simulink model "VB_RIFKF_GNSS_INS25"  (R2023a)
settings: Solver=FixedStepAuto  StartTime=0  StopTime=500  FixedStep=0.01  RelTol=1e-3
InitFcn:
  | resilient_initNavigation1216;
  | init_param;
undefined symbols (not defined in the file or in its folder): dt, g0, gam0_rad, ISUS_flag, magnitude, p, P0, P0_RIEKF, param, pd0, pe0, phi0_rad, pn0, psi, psi0_rad, state_dim, vd0, ve0, vn0
libraries: simulink_extras x68, dspstat3 x54, sharedtransform x47, simulink x43, matrix_library x9, sharedTrackingLibrary x5, dspfactors x4, aerolibconvert2 x3, aerolibtransform2 x3
(part 12 of 22)

== system VB_RIFKF_GNSS_INS25/No.1_Sensor_Data_Process1/GPS_Data_Process/LLA2NED ==
  note: Vecef2ned
  gps_LLA_rad : Inport
  GPSfixtype : Inport  Port=2
  GPS_Vecef_m/s : Inport  Port=3
  QGC_sensor_reinit : Inport  Port=4
  GPS0 : Inport  Port=5
  Angle Conversion1 : aerolibconvert2/Angle Conversion  IU=deg  OU=rad
  Bus Creator : BusCreator  Inputs=3
  Bus Creator1 : BusCreator  Inputs=3
  Bus Selector : BusSelector  OutputSignals=lon_gps,lat_gps
  Bus Selector1 : BusSelector  OutputSignals=lat_gps,lon_gps,H_gps
  Constant1 : Constant  Value=-90
  Constant4 : Constant  Value=0
  Data Type Conversion{,1..3} (4 alike) : DataTypeConversion  OutDataTypeStr=single  SaturateOnIntegerOverflow=off  RndMeth=Floor
  Demux : Demux  Outputs=3
  Demux1 : Demux  Outputs=3
  Demux3 : Demux  Outputs=3
  Detect Increase : simulink/Logic and Bit Operations/Detect Increase  vinit=0.0  OutDataTypeStr=boolean
  Digital Clock : DigitalClock  SampleTime=0.01
  Direction Cosine Matrix ECEF to NED : aerolibtransform2/Direction Cosine Matrix ECEF to NED  Commented=on
  Divide1 : Product  Inputs=**  Multiplication=Matrix(*)
  Gain : Gain  Gain=-1
  LLA to ECEF Position : LLA2ECEF  R=6378137
  LLA to ECEF Position1 : LLA2ECEF  R=6378137
  MATLAB Function2 : MATLAB Function  TreatAsAtomicUnit=on
  Mux2 : Mux  Inputs=3
  Mux5 : Mux  Inputs=2
  Mux6 : Mux  Inputs=2
  Product : Product  Commented=on  Multiplication=Matrix(*)
  Radians to Degrees{,1..3} (4 alike) : simulink_extras/Transformations/Radians to Degrees
  Radians to Degrees4 : simulink_extras/Transformations/Radians to Degrees  Commented=on
  Rotation Angles to Direction Cosine Matrix : sharedtransform/Rotation Angles to Direction Cosine Matrix  rotationOrder=ZYX  aMode=aMode
  Scope1 : Scope
  Selector2 : Selector  Commented=on  InputPortWidth=3  IndexOptions=Index vector (dialog)  Indices=[1 2]  OutputSizes=1
  Sum : Sum  Inputs=|++
  Sum1 : Sum  Inputs=|+-
  initGPSLLA : MATLAB Function  TreatAsAtomicUnit=on
  "gpsposNEDout " : Outport
  gpsvNEDout : Outport  Port=2
  wires:
  GPSfixtype/1 -> initGPSLLA/2(GPSfixtype)
  Bus Creator1/1 -> "gpsposNEDout "/1, Scope1/1
  Demux3/3 -> Data Type Conversion2/1  "gpspos_D"
  Demux3/2 -> Data Type Conversion1/1  "gpspos_E"
  Demux3/1 -> Data Type Conversion/1  "gpspos_N"
  Bus Creator/1 -> Bus Selector/1, Bus Selector1/1
  Demux/3 -> Bus Creator/3  "H_gps"
  Demux/2 -> Bus Creator/2  "lon_gps"
  Demux/1 -> Bus Creator/1  "lat_gps"
  Demux1/3 -> LLA to ECEF Position1/2
  Mux6/1 -> LLA to ECEF Position1/1
  Mux5/1 -> LLA to ECEF Position/1
  Gain/1 -> Sum/1
  LLA to ECEF Position1/1 -> Sum1/1
  Constant4/1 -> Mux2/3
  Sum1/1 -> Divide1/2
  Demux1/1 -> Radians to Degrees/1
  Mux2/1 -> Rotation Angles to Direction Cosine Matrix/1
  Rotation Angles to Direction Cosine Matrix/1 -> Divide1/1
  Constant1/1 -> Angle Conversion1/1
  LLA to ECEF Position/1 -> Sum1/2
  Demux1/2 -> Radians to Degrees1/1
  Sum/1 -> Mux2/2
  Bus Selector/2 -> Gain/1  "<lat_gps>"
  Bus Selector/1 -> Mux2/1  "<lon_gps>"
  Bus Selector1/1 -> Radians to Degrees2/1  "<lat_gps>"
  Bus Selector1/2 -> Radians to Degrees3/1  "<lon_gps>"
  Bus Selector1/3 -> LLA to ECEF Position/2  "<H_gps>"
  gps_LLA_rad/1 -> initGPSLLA/3(gps_LLA_rad), Selector2/1, Demux1/1
  Radians to Degrees/1 -> Mux6/1
  Radians to Degrees1/1 -> Mux6/2
  QGC_sensor_reinit/1 -> Detect Increase/1
  Data Type Conversion/1 -> Bus Creator1/1  "gpspos_N"
  Data Type Conversion1/1 -> Bus Creator1/2  "gpspos_E"
  Data Type Conversion2/1 -> Bus Creator1/3  "gpspos_D"
  Angle Conversion1/1 -> Sum/2
  Radians to Degrees2/1 -> Mux5/1
  Radians to Degrees3/1 -> Mux5/2
  GPS_Vecef_m/s/1 -> Data Type Conversion3/1, Product/2
  Direction Cosine Matrix ECEF to NED/1 -> Product/1
  Selector2/1 -> Radians to Degrees4/1
  Radians to Degrees4/1 -> Direction Cosine Matrix ECEF to NED/1
  Data Type Conversion3/1 -> gpsvNEDout/1  "gpspos_N"
  Detect Increase/1 -> initGPSLLA/1(QGCinitflag)
  initGPSLLA/1(gpsLLA0_rad) -> Demux/1
  Divide1/1 -> Demux3/1, MATLAB Function2/2(u)
  Digital Clock/1 -> MATLAB Function2/1(t)

== system VB_RIFKF_GNSS_INS25/No.1_Sensor_Data_Process1/GPS_Data_Process/heading_GPS ==
  Vned : Inport
  Atan2 : Trigonometry  Operator=atan2
  Compare To Constant : simulink/Logic and Bit Operations/Compare To Constant  relop=>=  const=0.8  OutDataTypeStr=boolean
  Math Function : Math  Operator=magnitude^2  SignedPower=on
  Moving Average1 : dspstat3/Moving Average  Commented=on  Method=Sliding window  ForgettingFactorPort=off  SpecifyWindowLength=on  WindowLength=10  OverlapLength=9  AllowArbitraryInputLength=off  ForgettingFactor=0.9  SimulateUsing=Code generation
  Scope : Scope  NumInputPorts=2
  Scope1 : Scope
  Selector2 : Selector  InputPortWidth=3  IndexOptions=Index vector (dialog)  Indices=[2]  OutputSizes=1
  Selector3 : Selector  InputPortWidth=3  IndexOptions=Index vector (dialog)  Indices=[1]  OutputSizes=1
  Selector4 : Selector  InputPortWidth=3  IndexOptions=Index vector (dialog)  Indices=[1 2]  OutputSizes=1
  Sqrt : Sqrt
  Sum of Elements : Sum  Inputs=+
  heading_GPS_rad : Outport
  heading_GPS_valid : Outport  Port=2
  wires:
  Selector2/1 -> Atan2/1
  Math Function/1 -> Sum of Elements/1
  Vned/1 -> Selector2/1, Selector4/1, Selector3/1
  Selector3/1 -> Atan2/2
  Sum of Elements/1 -> Sqrt/1
  Selector4/1 -> Math Function/1
  Sqrt/1 -> Compare To Constant/1
  Compare To Constant/1 -> Scope1/1, heading_GPS_valid/1
  Atan2/1 -> Scope/1, Scope/2, heading_GPS_rad/1

== system VB_RIFKF_GNSS_INS25/No.1_Sensor_Data_Process1/IMU_Data_Process/Bias Eliminate ==
  gyro_B_rad/s_ori : Inport
  Data Type Conversion : DataTypeConversion  OutDataTypeStr=single  SaturateOnIntegerOverflow=off  RndMeth=Floor
  Digital Clock : DigitalClock
  Memory : Memory
  Scope : Scope
  Subsystem : Subsystem
  Sum : Sum  Inputs=|+-
  Switch : Switch  Criteria=u2 > Threshold  Threshold=5  SaturateOnIntegerOverflow=off  InputSameDT=off
  Out1 : Outport
  wires:
  Data Type Conversion/1 -> Out1/1
  gyro_B_rad/s_ori/1 -> Subsystem/1(data), Sum/1
  Sum/1 -> Data Type Conversion/1
  Digital Clock/1 -> Switch/2
  Subsystem/1(mean_data) -> Switch/3
  Switch/1 -> Scope/1, Memory/1
  Memory/1 -> Switch/1

== system VB_RIFKF_GNSS_INS25/No.1_Sensor_Data_Process1/IMU_Data_Process/accl_preprocessing2 ==
  note: front-right-dowm
  accl_B_m/s_ori : Inport
  Constant2 : Constant  Value=1/dt  OutDataTypeStr=single
  Constant4 : Constant  Value=1/dt  OutDataTypeStr=single
  Constant6 : Constant  Value=1/dt  OutDataTypeStr=single
  Constant7 : Constant  Value=param.proces.imu_gyro_cutoff_freq  OutDataTypeStr=single
  Demux : Demux  Outputs=3
  MATLAB Function1 : MATLAB Function  TreatAsAtomicUnit=on
  MATLAB Function2 : MATLAB Function  TreatAsAtomicUnit=on
  MATLAB Function3 : MATLAB Function  TreatAsAtomicUnit=on
  Vector Concatenate : Concatenate  NumInputs=3
  accl_B_m/s2_LPF : Outport
  wires:
  Vector Concatenate/1 -> accl_B_m/s2_LPF/1
  Constant4/1 -> MATLAB Function2/2(sample_freq)
  Constant2/1 -> MATLAB Function1/2(sample_freq)
  accl_B_m/s_ori/1 -> Demux/1
  Demux/1 -> MATLAB Function2/1(curr_input)
  Demux/2 -> MATLAB Function1/1(curr_input)
  Constant6/1 -> MATLAB Function3/2(sample_freq)
  Demux/3 -> MATLAB Function3/1(curr_input)
  Constant7/1 -> MATLAB Function2/3(cutoff_freq), MATLAB Function3/3(cutoff_freq), MATLAB Function1/3(cutoff_freq)
  MATLAB Function3/1(curr_output) -> Vector Concatenate/3  "wz"
  MATLAB Function1/1(curr_output) -> Vector Concatenate/2  "wy"
  MATLAB Function2/1(curr_output) -> Vector Concatenate/1  "wx"

== system VB_RIFKF_GNSS_INS25/No.1_Sensor_Data_Process1/IMU_Data_Process/gyro_preprocessing2 ==
  note: front-right-dowm
  note: rad/s
  gyro_B_rad/s_ori : Inport
  Constant2 : Constant  Value=1/dt  OutDataTypeStr=single
  Constant4 : Constant  Value=1/dt  OutDataTypeStr=single
  Constant6 : Constant  Value=1/dt  OutDataTypeStr=single
  Constant7 : Constant  Value=param.proces.imu_gyro_cutoff_freq  OutDataTypeStr=single
  Demux : Demux  Outputs=3
  MATLAB Function1 : MATLAB Function  TreatAsAtomicUnit=on
  MATLAB Function2 : MATLAB Function  TreatAsAtomicUnit=on
  MATLAB Function3 : MATLAB Function  TreatAsAtomicUnit=on
  Scope : Scope  NumInputPorts=2
  Vector Concatenate : Concatenate  NumInputs=3
  gyro_B_rad/s_LPF : Outport  PortDimensions=3
  wires:
  MATLAB Function2/1(curr_output) -> Vector Concatenate/1  "wx"
  MATLAB Function1/1(curr_output) -> Vector Concatenate/2  "wy"
  MATLAB Function3/1(curr_output) -> Vector Concatenate/3  "wz"
  Constant7/1 -> MATLAB Function3/3(cutoff_freq), MATLAB Function1/3(cutoff_freq), MATLAB Function2/3(cutoff_freq)
  Demux/3 -> MATLAB Function3/1(curr_input)
  Constant6/1 -> MATLAB Function3/2(sample_freq)
  Demux/2 -> MATLAB Function1/1(curr_input)
  Demux/1 -> MATLAB Function2/1(curr_input), Scope/2
  gyro_B_rad/s_ori/1 -> Demux/1
  Constant2/1 -> MATLAB Function1/2(sample_freq)
  Constant4/1 -> MATLAB Function2/2(sample_freq)
  Vector Concatenate/1 -> gyro_B_rad/s_LPF/1

== system VB_RIFKF_GNSS_INS25/No.1_Sensor_Data_Process1/Magn_Data_Process/Magn_preprocessing ==
  note: front-right-dowm
  Magn_B_rad/s_ori : Inport
  Constant2 : Constant  Value=1/dt  OutDataTypeStr=single
  Constant4 : Constant  Value=1/dt  OutDataTypeStr=single
  Constant6 : Constant  Value=1/dt  OutDataTypeStr=single
  Constant7 : Constant  Value=param.proces.imu_gyro_cutoff_freq  OutDataTypeStr=single
  Demux : Demux  Outputs=3
  MATLAB Function1 : MATLAB Function  TreatAsAtomicUnit=on
  MATLAB Function2 : MATLAB Function  TreatAsAtomicUnit=on
  MATLAB Function3 : MATLAB Function  TreatAsAtomicUnit=on
  Scope : Scope  NumInputPorts=2
  Vector Concatenate : Concatenate  NumInputs=3
  Magn_B_rad/s_LPF : Outport
  wires:
  Vector Concatenate/1 -> Magn_B_rad/s_LPF/1
  Constant4/1 -> MATLAB Function2/2(sample_freq)
  Constant2/1 -> MATLAB Function1/2(sample_freq)
  Magn_B_rad/s_ori/1 -> Demux/1
  Demux/1 -> Scope/2, MATLAB Function2/1(curr_input)
  Demux/2 -> MATLAB Function1/1(curr_input)
  Constant6/1 -> MATLAB Function3/2(sample_freq)
  Demux/3 -> MATLAB Function3/1(curr_input)
  Constant7/1 -> MATLAB Function2/3(cutoff_freq), MATLAB Function1/3(cutoff_freq), MATLAB Function3/3(cutoff_freq)
  MATLAB Function3/1(curr_output) -> Vector Concatenate/3  "wz"
  MATLAB Function1/1(curr_output) -> Vector Concatenate/2  "wy"
  MATLAB Function2/1(curr_output) -> Vector Concatenate/1  "wx"

== system VB_RIFKF_GNSS_INS25/No.1_Sensor_Data_Process1/Subsystem/TD_baro ==
  H_baro : Inport
  Constant1 : Constant  Value=dt  OutDataTypeStr=single
  Constant3 : Constant  Value=0.1  OutDataTypeStr=single
  Constant4 : Constant  Value=900  OutDataTypeStr=single
  Delay1 : Delay  DelayLength=1  InitialConditionSource=Input port
      settings: InputPortMap=u0,p4
  MATLAB Function2 : MATLAB Function  TreatAsAtomicUnit=on
  Memory : Memory  InheritSampleTime=on
  Scope : Scope  NumInputPorts=3
  vH_baro_TD : Outport
  H_baro_TD : Outport  Port=2
  wires:
  Delay1/1 -> H_baro_TD/1, Scope/3, MATLAB Function2/3("u1 ")
  H_baro/1 -> Delay1/2, MATLAB Function2/2(u0), Scope/1
  Memory/1 -> MATLAB Function2/4("u2 "), vH_baro_TD/1, Scope/2
  Constant3/1 -> MATLAB Function2/5(h)
  Constant1/1 -> MATLAB Function2/1(T)
  Constant4/1 -> MATLAB Function2/6(r)
  MATLAB Function2/1(u1) -> Delay1/1
  MATLAB Function2/2(u2) -> Memory/1

== system VB_RIFKF_GNSS_INS25/No.1_Sensor_Data_Process1/TOF_Data_Process/TD_baro ==
  H_TOF : Inport
  Constant1 : Constant  Value=dt  OutDataTypeStr=single
  Constant3 : Constant  Value=0.04  OutDataTypeStr=single
  Constant4 : Constant  Value=600  OutDataTypeStr=single
  Delay1 : Delay  DelayLength=1  InitialConditionSource=Input port
      settings: InputPortMap=u0,p4
  MATLAB Function2 : MATLAB Function  TreatAsAtomicUnit=on
  Memory : Memory  InheritSampleTime=on
  Scope : Scope  NumInputPorts=3
  vH_TOF_TD : Outport
  H_TOF_TD : Outport  Port=2
  wires:
  Delay1/1 -> H_TOF_TD/1, Scope/3, MATLAB Function2/3("u1 ")
  H_TOF/1 -> Delay1/2, MATLAB Function2/2(u0), Scope/1
  Memory/1 -> MATLAB Function2/4("u2 "), vH_TOF_TD/1, Scope/2
  Constant3/1 -> MATLAB Function2/5(h)
  Constant1/1 -> MATLAB Function2/1(T)
  Constant4/1 -> MATLAB Function2/6(r)
  MATLAB Function2/1(u1) -> Delay1/1
  MATLAB Function2/2(u2) -> Memory/1

== system VB_RIFKF_GNSS_INS25/No.1_Sensor_Data_Process1/TOF_Data_Process/reinit_TOF ==
  QGC_sensor_reinit : Inport
  Data : Inport  Port=2
  Detect Increase : simulink/Logic and Bit Operations/Detect Increase  vinit=0.0  OutDataTypeStr=boolean
  Switch : Switch  Criteria=u2 > Threshold  SaturateOnIntegerOverflow=off  InputSameDT=off
  Unit Delay : UnitDelay  SampleTime=-1  HasFrameUpgradeWarning=on
  dataout : Outport
  wires:
  Unit Delay/1 -> Switch/3
  Data/1 -> Switch/1
  Switch/1 -> dataout/1, Unit Delay/1
  Detect Increase/1 -> Switch/2
  QGC_sensor_reinit/1 -> Detect Increase/1

== system VB_RIFKF_GNSS_INS25/No.1_Sensor_Data_Process1/baro_Data_Process/Pressure2Height ==
  baro : Inport
  Add : Sum  Inputs=+-
  Constant : Constant  OutDataTypeStr=single
  Constant1 : Constant  Value=1/5.255  OutDataTypeStr=single
  Gain : Gain  Gain=1/1.01325
  Gain1 : Gain  Gain=44330
  Math Function : Math  Operator=pow  SignedPower=on
  H_baro : Outport
  wires:
  Gain/1 -> Math Function/1
  Constant1/1 -> Math Function/2
  Math Function/1 -> Add/2
  Constant/1 -> Add/1
  Add/1 -> Gain1/1
  Gain1/1 -> H_baro/1
  baro/1 -> Gain/1

== system VB_RIFKF_GNSS_INS25/No.1_Sensor_Data_Process1/baro_Data_Process/TD_baro ==
  H_baro : Inport
  Constant1 : Constant  Value=dt  OutDataTypeStr=single
  Constant3 : Constant  Value=0.23  OutDataTypeStr=single
  Constant4 : Constant  Value=900  OutDataTypeStr=single
  Delay1 : Delay  DelayLength=1  InitialConditionSource=Input port
      settings: InputPortMap=u0,p4
  MATLAB Function2 : MATLAB Function  TreatAsAtomicUnit=on
  Memory : Memory  InheritSampleTime=on
  Scope : Scope  NumInputPorts=3
  vH_baro_TD : Outport
  H_baro_TD : Outport  Port=2
  wires:
  Delay1/1 -> H_baro_TD/1, Scope/3, MATLAB Function2/3("u1 ")
  H_baro/1 -> Delay1/2, MATLAB Function2/2(u0), Scope/1
  Memory/1 -> MATLAB Function2/4("u2 "), vH_baro_TD/1, Scope/2
  Constant3/1 -> MATLAB Function2/5(h)
  Constant1/1 -> MATLAB Function2/1(T)
  Constant4/1 -> MATLAB Function2/6(r)
  MATLAB Function2/1(u1) -> Delay1/1
  MATLAB Function2/2(u2) -> Memory/1

== system VB_RIFKF_GNSS_INS25/No.1_Sensor_Data_Process1/baro_Data_Process/TemCompensate1 ==
  baro_tem : Inport
  Add : Sum  Inputs=+++
  Constant2 : Constant  Value=-1663  OutDataTypeStr=single
  Gain : Gain  Gain=-1.6
  Gain1 : Gain  Gain=102.5
  Product : Product
  bias : Outport
  wires:
  Gain1/1 -> Add/2
  Add/1 -> bias/1
  Gain/1 -> Add/1
  Product/1 -> Gain/1
  Constant2/1 -> Add/3
  baro_tem/1 -> Product/1, Product/2, Gain1/1

== system VB_RIFKF_GNSS_INS25/No.1_Sensor_Data_Process1/baro_Data_Process/reinit_baro0 ==
  QGC_sensor_reinit : Inport
  Data : Inport  Port=2
  Detect Increase : simulink/Logic and Bit Operations/Detect Increase  vinit=0.0  OutDataTypeStr=boolean
  Switch : Switch  Criteria=u2 > Threshold  SaturateOnIntegerOverflow=off  InputSameDT=off
  Unit Delay : UnitDelay  SampleTime=-1  HasFrameUpgradeWarning=on
  dataout : Outport
  wires:
  Unit Delay/1 -> Switch/3
  Data/1 -> Switch/1
  Switch/1 -> dataout/1, Unit Delay/1
  Detect Increase/1 -> Switch/2
  QGC_sensor_reinit/1 -> Detect Increase/1

== system VB_RIFKF_GNSS_INS25/No.1_Sensor_Data_Process1/baro_Data_Process/reinit_baro1 ==
  QGC_sensor_reinit : Inport
  Data : Inport  Port=2
  Detect Increase : simulink/Logic and Bit Operations/Detect Increase  vinit=0.0  OutDataTypeStr=boolean
  Switch : Switch  Criteria=u2 > Threshold  SaturateOnIntegerOverflow=off  InputSameDT=off
  Unit Delay : UnitDelay  SampleTime=-1  HasFrameUpgradeWarning=on
  dataout : Outport
  wires:
  QGC_sensor_reinit/1 -> Detect Increase/1
  Detect Increase/1 -> Switch/2
  Switch/1 -> Unit Delay/1, dataout/1
  Data/1 -> Switch/1
  Unit Delay/1 -> Switch/3

== system VB_RIFKF_GNSS_INS25/No.1_Sensor_Data_Process2/GPS_Data_Process/LLA2NED ==
  note: Vecef2ned
  gps_LLA_rad : Inport
  GPSfixtype : Inport  Port=2
  GPS_Vecef_m/s : Inport  Port=3
  QGC_sensor_reinit : Inport  Port=4
  GPS0 : Inport  Port=5
  Angle Conversion1 : aerolibconvert2/Angle Conversion  IU=deg  OU=rad
  Bus Creator : BusCreator  Inputs=3
  Bus Creator1 : BusCreator  Inputs=3
  Bus Selector : BusSelector  OutputSignals=lon_gps,lat_gps
  Bus Selector1 : BusSelector  OutputSignals=lat_gps,lon_gps,H_gps
  Constant1 : Constant  Value=-90
  Constant4 : Constant  Value=0
  Data Type Conversion{,1..3} (4 alike) : DataTypeConversion  OutDataTypeStr=single  SaturateOnIntegerOverflow=off  RndMeth=Floor
  Demux : Demux  Outputs=3
  Demux1 : Demux  Outputs=3
  Demux3 : Demux  Outputs=3
  Detect Increase : simulink/Logic and Bit Operations/Detect Increase  vinit=0.0  OutDataTypeStr=boolean
  Direction Cosine Matrix ECEF to NED : aerolibtransform2/Direction Cosine Matrix ECEF to NED  Commented=on
  Divide1 : Product  Inputs=**  Multiplication=Matrix(*)
  Gain : Gain  Gain=-1
  LLA to ECEF Position : LLA2ECEF  R=6378137
  LLA to ECEF Position1 : LLA2ECEF  R=6378137
  Mux2 : Mux  Inputs=3
  Mux5 : Mux  Inputs=2
  Mux6 : Mux  Inputs=2
  Product : Product  Commented=on  Multiplication=Matrix(*)
  Radians to Degrees{,1..3} (4 alike) : simulink_extras/Transformations/Radians to Degrees
  Radians to Degrees4 : simulink_extras/Transformations/Radians to Degrees  Commented=on
  Rotation Angles to Direction Cosine Matrix : sharedtransform/Rotation Angles to Direction Cosine Matrix  rotationOrder=ZYX  aMode=aMode
  Scope1 : Scope
  Selector2 : Selector  Commented=on  InputPortWidth=3  IndexOptions=Index vector (dialog)  Indices=[1 2]  OutputSizes=1
  Sum : Sum  Inputs=|++
  Sum1 : Sum  Inputs=|+-
  initGPSLLA : MATLAB Function  TreatAsAtomicUnit=on
  "gpsposNEDout " : Outport
  gpsvNEDout : Outport  Port=2
  wires:
  initGPSLLA/1(gpsLLA0_rad) -> Demux/1
  Detect Increase/1 -> initGPSLLA/1(QGCinitflag)
  Data Type Conversion3/1 -> gpsvNEDout/1  "gpspos_N"
  Radians to Degrees4/1 -> Direction Cosine Matrix ECEF to NED/1
  Selector2/1 -> Radians to Degrees4/1
  Direction Cosine Matrix ECEF to NED/1 -> Product/1
  GPS_Vecef_m/s/1 -> Product/2, Data Type Conversion3/1
  Radians to Degrees3/1 -> Mux5/2
  Radians to Degrees2/1 -> Mux5/1
  Angle Conversion1/1 -> Sum/2
  Data Type Conversion2/1 -> Bus Creator1/3  "gpspos_D"
  Data Type Conversion1/1 -> Bus Creator1/2  "gpspos_E"
  Data Type Conversion/1 -> Bus Creator1/1  "gpspos_N"
  QGC_sensor_reinit/1 -> Detect Increase/1
  Radians to Degrees1/1 -> Mux6/2
  Radians to Degrees/1 -> Mux6/1
  gps_LLA_rad/1 -> Demux1/1, Selector2/1, initGPSLLA/3(gps_LLA_rad)
  Bus Selector1/3 -> LLA to ECEF Position/2  "<H_gps>"
  Bus Selector1/2 -> Radians to Degrees3/1  "<lon_gps>"
  Bus Selector1/1 -> Radians to Degrees2/1  "<lat_gps>"
  Bus Selector/1 -> Mux2/1  "<lon_gps>"
  Bus Selector/2 -> Gain/1  "<lat_gps>"
  Sum/1 -> Mux2/2
  Demux1/2 -> Radians to Degrees1/1
  LLA to ECEF Position/1 -> Sum1/2
  Constant1/1 -> Angle Conversion1/1
  Rotation Angles to Direction Cosine Matrix/1 -> Divide1/1
  Mux2/1 -> Rotation Angles to Direction Cosine Matrix/1
  Demux1/1 -> Radians to Degrees/1
  Divide1/1 -> Demux3/1
  Sum1/1 -> Divide1/2
  Constant4/1 -> Mux2/3
  LLA to ECEF Position1/1 -> Sum1/1
  Gain/1 -> Sum/1
  Mux5/1 -> LLA to ECEF Position/1
  Mux6/1 -> LLA to ECEF Position1/1
  Demux1/3 -> LLA to ECEF Position1/2
  Demux/1 -> Bus Creator/1  "lat_gps"
  Demux/2 -> Bus Creator/2  "lon_gps"
  Demux/3 -> Bus Creator/3  "H_gps"
  Bus Creator/1 -> Bus Selector/1, Bus Selector1/1
  Demux3/1 -> Data Type Conversion/1  "gpspos_N"
  Demux3/2 -> Data Type Conversion1/1  "gpspos_E"
  Demux3/3 -> Data Type Conversion2/1  "gpspos_D"
  Bus Creator1/1 -> Scope1/1, "gpsposNEDout "/1
  GPSfixtype/1 -> initGPSLLA/2(GPSfixtype)

== system VB_RIFKF_GNSS_INS25/No.1_Sensor_Data_Process2/GPS_Data_Process/heading_GPS ==
  Vned : Inport
  Atan2 : Trigonometry  Operator=atan2
  Compare To Constant : simulink/Logic and Bit Operations/Compare To Constant  relop=>=  const=0.8  OutDataTypeStr=boolean
  Math Function : Math  Operator=magnitude^2  SignedPower=on
  Moving Average1 : dspstat3/Moving Average  Commented=on  Method=Sliding window  ForgettingFactorPort=off  SpecifyWindowLength=on  WindowLength=10  OverlapLength=9  AllowArbitraryInputLength=off  ForgettingFactor=0.9  SimulateUsing=Code generation
  Scope : Scope  NumInputPorts=2
  Scope1 : Scope
  Selector2 : Selector  InputPortWidth=3  IndexOptions=Index vector (dialog)  Indices=[2]  OutputSizes=1
  Selector3 : Selector  InputPortWidth=3  IndexOptions=Index vector (dialog)  Indices=[1]  OutputSizes=1
  Selector4 : Selector  InputPortWidth=3  IndexOptions=Index vector (dialog)  Indices=[1 2]  OutputSizes=1
  Sqrt : Sqrt
  Sum of Elements : Sum  Inputs=+
  heading_GPS_rad : Outport
  heading_GPS_valid : Outport  Port=2
  wires:
  Atan2/1 -> heading_GPS_rad/1, Scope/2, Scope/1
  Compare To Constant/1 -> heading_GPS_valid/1, Scope1/1
  Sqrt/1 -> Compare To Constant/1
  Selector4/1 -> Math Function/1
  Sum of Elements/1 -> Sqrt/1
  Selector3/1 -> Atan2/2
  Vned/1 -> Selector3/1, Selector4/1, Selector2/1
  Math Function/1 -> Sum of Elements/1
  Selector2/1 -> Atan2/1

== system VB_RIFKF_GNSS_INS25/No.1_Sensor_Data_Process2/IMU_Data_Process/Bias Eliminate ==
  gyro_B_rad/s_ori : Inport
  Data Type Conversion : DataTypeConversion  OutDataTypeStr=single  SaturateOnIntegerOverflow=off  RndMeth=Floor
  Digital Clock : DigitalClock
  Memory : Memory
  Scope : Scope
  Subsystem : Subsystem
  Sum : Sum  Inputs=|+-
  Switch : Switch  Criteria=u2 > Threshold  Threshold=5  SaturateOnIntegerOverflow=off  InputSameDT=off
  Out1 : Outport
  wires:
  Memory/1 -> Switch/1
  Switch/1 -> Memory/1, Scope/1
  Subsystem/1(mean_data) -> Switch/3
  Digital Clock/1 -> Switch/2
  Sum/1 -> Data Type Conversion/1
  gyro_B_rad/s_ori/1 -> Sum/1, Subsystem/1(data)
  Data Type Conversion/1 -> Out1/1

== system VB_RIFKF_GNSS_INS25/No.1_Sensor_Data_Process2/IMU_Data_Process/accl_preprocessing2 ==
  note: front-right-dowm
  accl_B_m/s_ori : Inport
  Constant2 : Constant  Value=1/dt  OutDataTypeStr=single
  Constant4 : Constant  Value=1/dt  OutDataTypeStr=single
  Constant6 : Constant  Value=1/dt  OutDataTypeStr=single
  Constant7 : Constant  Value=param.proces.imu_gyro_cutoff_freq  OutDataTypeStr=single
  Demux : Demux  Outputs=3
  MATLAB Function1 : MATLAB Function  TreatAsAtomicUnit=on
  MATLAB Function2 : MATLAB Function  TreatAsAtomicUnit=on
  MATLAB Function3 : MATLAB Function  TreatAsAtomicUnit=on
  Vector Concatenate : Concatenate  NumInputs=3
  accl_B_m/s2_LPF : Outport
  wires:
  MATLAB Function2/1(curr_output) -> Vector Concatenate/1  "wx"
  MATLAB Function1/1(curr_output) -> Vector Concatenate/2  "wy"
  MATLAB Function3/1(curr_output) -> Vector Concatenate/3  "wz"
  Constant7/1 -> MATLAB Function1/3(cutoff_freq), MATLAB Function3/3(cutoff_freq), MATLAB Function2/3(cutoff_freq)
  Demux/3 -> MATLAB Function3/1(curr_input)
  Constant6/1 -> MATLAB Function3/2(sample_freq)
  Demux/2 -> MATLAB Function1/1(curr_input)
  Demux/1 -> MATLAB Function2/1(curr_input)
  accl_B_m/s_ori/1 -> Demux/1
  Constant2/1 -> MATLAB Function1/2(sample_freq)
  Constant4/1 -> MATLAB Function2/2(sample_freq)
  Vector Concatenate/1 -> accl_B_m/s2_LPF/1

== system VB_RIFKF_GNSS_INS25/No.1_Sensor_Data_Process2/IMU_Data_Process/gyro_preprocessing2 ==
  note: rad/s
  note: front-right-dowm
  gyro_B_rad/s_ori : Inport
  Constant2 : Constant  Value=1/dt  OutDataTypeStr=single
  Constant4 : Constant  Value=1/dt  OutDataTypeStr=single
  Constant6 : Constant  Value=1/dt  OutDataTypeStr=single
  Constant7 : Constant  Value=param.proces.imu_gyro_cutoff_freq  OutDataTypeStr=single
  Demux : Demux  Outputs=3
  MATLAB Function1 : MATLAB Function  TreatAsAtomicUnit=on
  MATLAB Function2 : MATLAB Function  TreatAsAtomicUnit=on
  MATLAB Function3 : MATLAB Function  TreatAsAtomicUnit=on
  Scope : Scope  NumInputPorts=2
  Vector Concatenate : Concatenate  NumInputs=3
  gyro_B_rad/s_LPF : Outport  PortDimensions=3
  wires:
  Vector Concatenate/1 -> gyro_B_rad/s_LPF/1
  Constant4/1 -> MATLAB Function2/2(sample_freq)
  Constant2/1 -> MATLAB Function1/2(sample_freq)
  gyro_B_rad/s_ori/1 -> Demux/1
  Demux/1 -> Scope/2, MATLAB Function2/1(curr_input)
  Demux/2 -> MATLAB Function1/1(curr_input)
  Constant6/1 -> MATLAB Function3/2(sample_freq)
  Demux/3 -> MATLAB Function3/1(curr_input)
  Constant7/1 -> MATLAB Function2/3(cutoff_freq), MATLAB Function1/3(cutoff_freq), MATLAB Function3/3(cutoff_freq)
  MATLAB Function3/1(curr_output) -> Vector Concatenate/3  "wz"
  MATLAB Function1/1(curr_output) -> Vector Concatenate/2  "wy"
  MATLAB Function2/1(curr_output) -> Vector Concatenate/1  "wx"

== system VB_RIFKF_GNSS_INS25/No.1_Sensor_Data_Process2/Magn_Data_Process/Magn_preprocessing ==
  note: front-right-dowm
  Magn_B_rad/s_ori : Inport
  Constant2 : Constant  Value=1/dt  OutDataTypeStr=single
  Constant4 : Constant  Value=1/dt  OutDataTypeStr=single
  Constant6 : Constant  Value=1/dt  OutDataTypeStr=single
  Constant7 : Constant  Value=param.proces.imu_gyro_cutoff_freq  OutDataTypeStr=single
  Demux : Demux  Outputs=3
  MATLAB Function1 : MATLAB Function  TreatAsAtomicUnit=on
  MATLAB Function2 : MATLAB Function  TreatAsAtomicUnit=on
  MATLAB Function3 : MATLAB Function  TreatAsAtomicUnit=on
  Scope : Scope  NumInputPorts=2
  Vector Concatenate : Concatenate  NumInputs=3
  Magn_B_rad/s_LPF : Outport
  wires:
  MATLAB Function2/1(curr_output) -> Vector Concatenate/1  "wx"
  MATLAB Function1/1(curr_output) -> Vector Concatenate/2  "wy"
  MATLAB Function3/1(curr_output) -> Vector Concatenate/3  "wz"
  Constant7/1 -> MATLAB Function3/3(cutoff_freq), MATLAB Function1/3(cutoff_freq), MATLAB Function2/3(cutoff_freq)
  Demux/3 -> MATLAB Function3/1(curr_input)
  Constant6/1 -> MATLAB Function3/2(sample_freq)
  Demux/2 -> MATLAB Function1/1(curr_input)
  Demux/1 -> MATLAB Function2/1(curr_input), Scope/2
  Magn_B_rad/s_ori/1 -> Demux/1
  Constant2/1 -> MATLAB Function1/2(sample_freq)
  Constant4/1 -> MATLAB Function2/2(sample_freq)
  Vector Concatenate/1 -> Magn_B_rad/s_LPF/1

== system VB_RIFKF_GNSS_INS25/No.1_Sensor_Data_Process2/Subsystem/TD_baro ==
  H_baro : Inport
  Constant1 : Constant  Value=dt  OutDataTypeStr=single
  Constant3 : Constant  Value=0.1  OutDataTypeStr=single
  Constant4 : Constant  Value=900  OutDataTypeStr=single
  Delay1 : Delay  DelayLength=1  InitialConditionSource=Input port
      settings: InputPortMap=u0,p4
  MATLAB Function2 : MATLAB Function  TreatAsAtomicUnit=on
  Memory : Memory  InheritSampleTime=on
  Scope : Scope  NumInputPorts=3
  vH_baro_TD : Outport
  H_baro_TD : Outport  Port=2
  wires:
  MATLAB Function2/2(u2) -> Memory/1
  MATLAB Function2/1(u1) -> Delay1/1
  Constant4/1 -> MATLAB Function2/6(r)
  Constant1/1 -> MATLAB Function2/1(T)
  Constant3/1 -> MATLAB Function2/5(h)
  Memory/1 -> Scope/2, vH_baro_TD/1, MATLAB Function2/4("u2 ")
  H_baro/1 -> Scope/1, MATLAB Function2/2(u0), Delay1/2
  Delay1/1 -> MATLAB Function2/3("u1 "), Scope/3, H_baro_TD/1

== system VB_RIFKF_GNSS_INS25/No.1_Sensor_Data_Process2/TOF_Data_Process/TD_baro ==
  H_TOF : Inport
  Constant1 : Constant  Value=dt  OutDataTypeStr=single
  Constant3 : Constant  Value=0.04  OutDataTypeStr=single
  Constant4 : Constant  Value=600  OutDataTypeStr=single
  Delay1 : Delay  DelayLength=1  InitialConditionSource=Input port
      settings: InputPortMap=u0,p4
  MATLAB Function2 : MATLAB Function  TreatAsAtomicUnit=on
  Memory : Memory  InheritSampleTime=on
  Scope : Scope  NumInputPorts=3
  vH_TOF_TD : Outport
  H_TOF_TD : Outport  Port=2
  wires:
  MATLAB Function2/2(u2) -> Memory/1
  MATLAB Function2/1(u1) -> Delay1/1
  Constant4/1 -> MATLAB Function2/6(r)
  Constant1/1 -> MATLAB Function2/1(T)
  Constant3/1 -> MATLAB Function2/5(h)
  Memory/1 -> Scope/2, vH_TOF_TD/1, MATLAB Function2/4("u2 ")
  H_TOF/1 -> Scope/1, MATLAB Function2/2(u0), Delay1/2
  Delay1/1 -> MATLAB Function2/3("u1 "), Scope/3, H_TOF_TD/1

== system VB_RIFKF_GNSS_INS25/No.1_Sensor_Data_Process2/TOF_Data_Process/reinit_TOF ==
  QGC_sensor_reinit : Inport
  Data : Inport  Port=2
  Detect Increase : simulink/Logic and Bit Operations/Detect Increase  vinit=0.0  OutDataTypeStr=boolean
  Switch : Switch  Criteria=u2 > Threshold  SaturateOnIntegerOverflow=off  InputSameDT=off
  Unit Delay : UnitDelay  SampleTime=-1  HasFrameUpgradeWarning=on
  dataout : Outport
  wires:
  QGC_sensor_reinit/1 -> Detect Increase/1
  Detect Increase/1 -> Switch/2
  Switch/1 -> Unit Delay/1, dataout/1
  Data/1 -> Switch/1
  Unit Delay/1 -> Switch/3

== system VB_RIFKF_GNSS_INS25/No.1_Sensor_Data_Process2/baro_Data_Process/Pressure2Height ==
  baro : Inport
  Add : Sum  Inputs=+-
  Constant : Constant  OutDataTypeStr=single
  Constant1 : Constant  Value=1/5.255  OutDataTypeStr=single
  Gain : Gain  Gain=1/1.01325
  Gain1 : Gain  Gain=44330
  Math Function : Math  Operator=pow  SignedPower=on
  H_baro : Outport
  wires:
  baro/1 -> Gain/1
  Gain1/1 -> H_baro/1
  Add/1 -> Gain1/1
  Constant/1 -> Add/1
  Math Function/1 -> Add/2
  Constant1/1 -> Math Function/2
  Gain/1 -> Math Function/1

== system VB_RIFKF_GNSS_INS25/No.1_Sensor_Data_Process2/baro_Data_Process/TD_baro ==
  H_baro : Inport
  Constant1 : Constant  Value=dt  OutDataTypeStr=single
  Constant3 : Constant  Value=0.23  OutDataTypeStr=single
  Constant4 : Constant  Value=900  OutDataTypeStr=single
  Delay1 : Delay  DelayLength=1  InitialConditionSource=Input port
      settings: InputPortMap=u0,p4
  MATLAB Function2 : MATLAB Function  TreatAsAtomicUnit=on
  Memory : Memory  InheritSampleTime=on
  Scope : Scope  NumInputPorts=3
  vH_baro_TD : Outport
  H_baro_TD : Outport  Port=2
  wires:
  MATLAB Function2/2(u2) -> Memory/1
  MATLAB Function2/1(u1) -> Delay1/1
  Constant4/1 -> MATLAB Function2/6(r)
  Constant1/1 -> MATLAB Function2/1(T)
  Constant3/1 -> MATLAB Function2/5(h)
  Memory/1 -> Scope/2, vH_baro_TD/1, MATLAB Function2/4("u2 ")
  H_baro/1 -> Scope/1, MATLAB Function2/2(u0), Delay1/2
  Delay1/1 -> MATLAB Function2/3("u1 "), Scope/3, H_baro_TD/1

== system VB_RIFKF_GNSS_INS25/No.1_Sensor_Data_Process2/baro_Data_Process/TemCompensate1 ==
  baro_tem : Inport
  Add : Sum  Inputs=+++
  Constant2 : Constant  Value=-1663  OutDataTypeStr=single
  Gain : Gain  Gain=-1.6
  Gain1 : Gain  Gain=102.5
  Product : Product
  bias : Outport
  wires:
  baro_tem/1 -> Gain1/1, Product/2, Product/1
  Constant2/1 -> Add/3
  Product/1 -> Gain/1
  Gain/1 -> Add/1
  Add/1 -> bias/1
  Gain1/1 -> Add/2

== system VB_RIFKF_GNSS_INS25/No.1_Sensor_Data_Process2/baro_Data_Process/reinit_baro0 ==
  QGC_sensor_reinit : Inport
  Data : Inport  Port=2
  Detect Increase : simulink/Logic and Bit Operations/Detect Increase  vinit=0.0  OutDataTypeStr=boolean
  Switch : Switch  Criteria=u2 > Threshold  SaturateOnIntegerOverflow=off  InputSameDT=off
  Unit Delay : UnitDelay  SampleTime=-1  HasFrameUpgradeWarning=on
  dataout : Outport
  wires:
  QGC_sensor_reinit/1 -> Detect Increase/1
  Detect Increase/1 -> Switch/2
  Switch/1 -> Unit Delay/1, dataout/1
  Data/1 -> Switch/1
  Unit Delay/1 -> Switch/3

== system VB_RIFKF_GNSS_INS25/No.1_Sensor_Data_Process2/baro_Data_Process/reinit_baro1 ==
  QGC_sensor_reinit : Inport
  Data : Inport  Port=2
  Detect Increase : simulink/Logic and Bit Operations/Detect Increase  vinit=0.0  OutDataTypeStr=boolean
  Switch : Switch  Criteria=u2 > Threshold  SaturateOnIntegerOverflow=off  InputSameDT=off
  Unit Delay : UnitDelay  SampleTime=-1  HasFrameUpgradeWarning=on
  dataout : Outport
  wires:
  Unit Delay/1 -> Switch/3
  Data/1 -> Switch/1
  Switch/1 -> dataout/1, Unit Delay/1
  Detect Increase/1 -> Switch/2
  QGC_sensor_reinit/1 -> Detect Increase/1

== system VB_RIFKF_GNSS_INS25/ER EKF/Error State Kalman Filter/Extended Kalman Filter1/Correct1 ==
  yMeas : Inport  SampleTime=SampleTime
  R : Inport  Port=2  SampleTime=SampleTime
  uMeas : Inport  Port=3  SampleTime=SampleTime
  uBlockOrdering : Inport  Port=4  SampleTime=SampleTime
  Enable : EnablePort
  Cast To Double : DataTypeConversion  OutDataTypeStr=single  SaturateOnIntegerOverflow=off  RndMeth=Floor
  Cast To Double1 : DataTypeConversion  OutDataTypeStr=single  SaturateOnIntegerOverflow=off  RndMeth=Floor
  Constant : Constant
  Constant6 : Constant  Value=[eye(6),zeros(6,9)]  OutDataTypeStr=single
  Correct1 : MATLAB Function  TreatAsAtomicUnit=on
  Correct2 : MATLAB Function  Commented=on  TreatAsAtomicUnit=on
  Data Store ReadP : DataStoreRead  DataStoreName=P  IndexOptions=Index vector (dialog)  Indices=1  OutputSizes=1
  Data Store ReadX : DataStoreRead  DataStoreName=x  IndexOptions=Index vector (dialog)  Indices=1  OutputSizes=1
  Data Store WriteP : DataStoreWrite  DataStoreName=P  IndexOptions=Index vector (dialog)  Indices=1  OutputSizes=1
  Data Store WriteX : DataStoreWrite  DataStoreName=x  IndexOptions=Index vector (dialog)  Indices=1  OutputSizes=1
  Delay : Delay  DelayLength=1  InitialCondition=[1 1 1 1 1 1]
  Delay1 : Delay  DelayLength=1  InitialCondition=[0.1,0.1,0.1,0.1,0.1,0.1]
  Display : Display
  Display1 : Display
  MATLAB Function : MATLAB Function  TreatAsAtomicUnit=on
  RegisterSimulinkFcn : S-Function  FunctionName=ekfukfRegisterSimulinkFcn  Parameters=int32(3), 1, pM.HasAdditiveNoise, SampleTime, DataType, SLFcnsToRegister  SFunctionDeploymentMode=off  EnableBusSupport=off
  Scope : Scope
  Scope1 : Scope
  Sk_m_innovation : Subsystem
  yBlockOrdering : Outport  VectorParamsAs1DForOutWhenUnconnected=off
  wires:
  Data Store ReadX/1 -> Sk_m_innovation/3(X), Correct1/1(x), RegisterSimulinkFcn/1
  Data Store ReadP/1 -> Sk_m_innovation/1(Pk/k_1), Correct1/2("P ")
  Correct1/2(P) -> Data Store WriteP/1
  R/1 -> Sk_m_innovation/4(R), RegisterSimulinkFcn/3, Correct1/4("R ")
  Correct1/1(xNew) -> Data Store WriteX/1
  Correct1/3(blockOrdering) -> yBlockOrdering/1
  uBlockOrdering/1 -> Correct1/6("blockOrdering ")
  uMeas/1 -> Correct1/5(uMeas)
  yMeas/1 -> Sk_m_innovation/2(yMeas), RegisterSimulinkFcn/2, Correct1/3(yMeas)
  Sk_m_innovation/1(measurement innovation) -> Scope/1
  Constant/1 -> Correct1/9(N)
  Delay/1 -> Cast To Double1/1
  Correct1/5(beta) -> Delay1/1
  Delay1/1 -> Cast To Double/1
  Constant6/1 -> Correct1/10(H)
  Cast To Double/1 -> Correct1/8("beta ")
  Cast To Double1/1 -> Correct1/7("alfa ")
  Correct1/4(alfa) -> Delay/1
  Correct1/6(R_VB) -> MATLAB Function/1(R), Display/1
  Correct1/7(R) -> Display1/1
  MATLAB Function/1(diagonal_elements) -> Scope1/1

== system VB_RIFKF_GNSS_INS25/ER EKF/Error State Kalman Filter/Extended Kalman Filter1/Output ==
  uBlockOrdering : Inport
  Data Store Read : DataStoreRead  DataStoreName=x  IndexOptions=Index vector (dialog)  Indices=1  OutputSizes=1
  Data Store Read1 : DataStoreRead  DataStoreName=P  IndexOptions=Index vector (dialog)  Indices=1  OutputSizes=1
  MATLAB Function : MATLAB Function  TreatAsAtomicUnit=on
  x : Outport  VectorParamsAs1DForOutWhenUnconnected=off
  P : Outport  Port=2  VectorParamsAs1DForOutWhenUnconnected=off
  yBlockOrdering : Outport  Port=3  VectorParamsAs1DForOutWhenUnconnected=off
  wires:
  Data Store Read/1 -> x/1
  Data Store Read1/1 -> MATLAB Function/1(S)
  uBlockOrdering/1 -> yBlockOrdering/1
  MATLAB Function/1(P) -> P/1

== system VB_RIFKF_GNSS_INS25/ER EKF/Error State Kalman Filter/Extended Kalman Filter1/Predict ==
  Q : Inport  SampleTime=SampleTime
  uState : Inport  Port=2  SampleTime=SampleTime
  uBlockOrdering : Inport  Port=3  SampleTime=SampleTime
  Data Store Read1 : DataStoreRead  Commented=on  DataStoreName=feedback_flag_18dim  IndexOptions=Index vector (dialog)  Indices=1  OutputSizes=1
  Data Store Write : DataStoreWrite  DataStoreName=P  IndexOptions=Index vector (dialog)  Indices=1  OutputSizes=1
  Data Store Write1 : DataStoreWrite  DataStoreName=x  IndexOptions=Index vector (dialog)  Indices=1  OutputSizes=1
  Data Store WriteX : DataStoreWrite  DataStoreName=x  IndexOptions=Index vector (dialog)  Indices=1  OutputSizes=1
  Data Store ReadP : DataStoreRead  DataStoreName=P  IndexOptions=Index vector (dialog)  Indices=1  OutputSizes=1
  Data Store ReadX : DataStoreRead  DataStoreName=x  IndexOptions=Index vector (dialog)  Indices=1  OutputSizes=1
  If : If  Commented=on  IfExpression=u1 == 1  ShowElse=off
  If Action Subsystem : Subsystem  Commented=on  TreatAsAtomicUnit=on
  Predict : MATLAB Function  TreatAsAtomicUnit=on
  RegisterSimulinkFcn : S-Function  FunctionName=ekfukfRegisterSimulinkFcn  Parameters=int32(2), 0, pS.HasAdditiveNoise, SampleTime, DataType, SLFcnsToRegister  SFunctionDeploymentMode=off  EnableBusSupport=off
  Zero : Constant  Value=zeros(15,1)  OutDataTypeStr=Inherit: Inherit via back propagation
  wires:
  Data Store ReadP/1 -> Predict/2("P ")
  Predict/2(P) -> Data Store Write/1
  Q/1 -> Predict/3(Q), RegisterSimulinkFcn/2
  Predict/1(xNew) -> Data Store WriteX/1
  Data Store ReadX/1 -> Predict/1(x), RegisterSimulinkFcn/1
  uBlockOrdering/1 -> Predict/5(unused)
  uState/1 -> Predict/4(uState)
  Data Store Read1/1 -> If/1
  If/1 -> If Action Subsystem/Action
  Zero/1 -> Data Store Write1/1

== system VB_RIFKF_GNSS_INS25/ER EKF/Error State Kalman Filter/Extended Kalman Filter2/Correct1 ==
  yMeas : Inport  SampleTime=SampleTime
  R : Inport  Port=2  SampleTime=SampleTime
  uMeas : Inport  Port=3  SampleTime=SampleTime
  uBlockOrdering : Inport  Port=4  SampleTime=SampleTime
  Enable : EnablePort
  Correct : MATLAB Function  TreatAsAtomicUnit=on
  Data Store ReadP : DataStoreRead  DataStoreName=P  IndexOptions=Index vector (dialog)  Indices=1  OutputSizes=1
  Data Store ReadX : DataStoreRead  DataStoreName=x  IndexOptions=Index vector (dialog)  Indices=1  OutputSizes=1
  Data Store WriteP : DataStoreWrite  DataStoreName=P  IndexOptions=Index vector (dialog)  Indices=1  OutputSizes=1
  Data Store WriteX : DataStoreWrite  DataStoreName=x  IndexOptions=Index vector (dialog)  Indices=1  OutputSizes=1
  RegisterSimulinkFcn : S-Function  FunctionName=ekfukfRegisterSimulinkFcn  Parameters=int32(3), 1, pM.HasAdditiveNoise, SampleTime, DataType, SLFcnsToRegister  SFunctionDeploymentMode=off  EnableBusSupport=off
  Scope : Scope
  Sk_m_innovation : Subsystem
  yBlockOrdering : Outport  VectorParamsAs1DForOutWhenUnconnected=off
  wires:
  Data Store ReadX/1 -> Sk_m_innovation/3(X), RegisterSimulinkFcn/1, Correct/1(x)
  Data Store ReadP/1 -> Sk_m_innovation/1(Pk/k_1), Correct/2("P ")
  Correct/2(P) -> Data Store WriteP/1
  R/1 -> Sk_m_innovation/4(R), Correct/4(R), RegisterSimulinkFcn/3
  Correct/1(xNew) -> Data Store WriteX/1
  Correct/3(blockOrdering) -> yBlockOrdering/1
  uBlockOrdering/1 -> Correct/6("blockOrdering ")
  uMeas/1 -> Correct/5(uMeas)
  yMeas/1 -> Sk_m_innovation/2(yMeas), RegisterSimulinkFcn/2, Correct/3(yMeas)
  Sk_m_innovation/1(measurement innovation) -> Scope/1

== system VB_RIFKF_GNSS_INS25/ER EKF/Error State Kalman Filter/Extended Kalman Filter2/Output ==
  uBlockOrdering : Inport
  Data Store Read : DataStoreRead  DataStoreName=x  IndexOptions=Index vector (dialog)  Indices=1  OutputSizes=1
  Data Store Read1 : DataStoreRead  DataStoreName=P  IndexOptions=Index vector (dialog)  Indices=1  OutputSizes=1
  MATLAB Function : MATLAB Function  TreatAsAtomicUnit=on
  x : Outport  VectorParamsAs1DForOutWhenUnconnected=off
  P : Outport  Port=2  VectorParamsAs1DForOutWhenUnconnected=off
  yBlockOrdering : Outport  Port=3  VectorParamsAs1DForOutWhenUnconnected=off
  wires:
  Data Store Read/1 -> x/1
  Data Store Read1/1 -> MATLAB Function/1(S)
  uBlockOrdering/1 -> yBlockOrdering/1
  MATLAB Function/1(P) -> P/1

== system VB_RIFKF_GNSS_INS25/ER EKF/Error State Kalman Filter/Extended Kalman Filter2/Predict ==
  Q : Inport  SampleTime=SampleTime
  uState : Inport  Port=2  SampleTime=SampleTime
  uBlockOrdering : Inport  Port=3  SampleTime=SampleTime
  Data Store Read1 : DataStoreRead  Commented=on  DataStoreName=feedback_flag_18dim  IndexOptions=Index vector (dialog)  Indices=1  OutputSizes=1
  Data Store Write : DataStoreWrite  DataStoreName=P  IndexOptions=Index vector (dialog)  Indices=1  OutputSizes=1
  Data Store Write1 : DataStoreWrite  DataStoreName=x  IndexOptions=Index vector (dialog)  Indices=1  OutputSizes=1
  Data Store WriteX : DataStoreWrite  DataStoreName=x  IndexOptions=Index vector (dialog)  Indices=1  OutputSizes=1
  Data Store ReadP : DataStoreRead  DataStoreName=P  IndexOptions=Index vector (dialog)  Indices=1  OutputSizes=1
  Data Store ReadX : DataStoreRead  DataStoreName=x  IndexOptions=Index vector (dialog)  Indices=1  OutputSizes=1
  If : If  Commented=on  IfExpression=u1 == 1  ShowElse=off
  If Action Subsystem : Subsystem  Commented=on  TreatAsAtomicUnit=on
  Predict : MATLAB Function  TreatAsAtomicUnit=on
  RegisterSimulinkFcn : S-Function  FunctionName=ekfukfRegisterSimulinkFcn  Parameters=int32(2), 0, pS.HasAdditiveNoise, SampleTime, DataType, SLFcnsToRegister  SFunctionDeploymentMode=off  EnableBusSupport=off
  Zero : Constant  Value=zeros(15,1)  OutDataTypeStr=Inherit: Inherit via back propagation
  wires:
  Data Store ReadP/1 -> Predict/2("P ")
  Predict/2(P) -> Data Store Write/1
  Q/1 -> Predict/3(Q), RegisterSimulinkFcn/2
  Predict/1(xNew) -> Data Store WriteX/1
  Data Store ReadX/1 -> Predict/1(x), RegisterSimulinkFcn/1
  uBlockOrdering/1 -> Predict/5(unused)
  uState/1 -> Predict/4(uState)
  Data Store Read1/1 -> If/1
  If/1 -> If Action Subsystem/Action
  Zero/1 -> Data Store Write1/1

== system VB_RIFKF_GNSS_INS25/ER EKF/Error State Kalman Filter/Simulink Function - State Transition/Cal Phi ==
  <DCM_b_n> : Inport
  wxyz : Inport  Port=2
  axyz : Inport  Port=3
  Constant : Constant  Value=dt
  MATLAB Function1 : MATLAB Function  TreatAsAtomicUnit=on
  Transpose : Math  Operator=transpose
  Phi : Outport
  wires:
  <DCM_b_n>/1 -> Transpose/1
  MATLAB Function1/1(Phi) -> Phi/1
  wxyz/1 -> MATLAB Function1/3(wxyz)
  axyz/1 -> MATLAB Function1/1(axyz)
  Constant/1 -> MATLAB Function1/4(dt)
  Transpose/1 -> MATLAB Function1/2(Cnb)

== system VB_RIFKF_GNSS_INS25/ER EKF/Error State Kalman Filter/Simulink Function - State Transition Jacobian/Cal Phi1 ==
  <DCM_b_n> : Inport
  wxyz : Inport  Port=2
  axyz : Inport  Port=3
  Constant : Constant  Value=dt
  MATLAB Function1 : MATLAB Function  TreatAsAtomicUnit=on
  Transpose : Math  Operator=transpose
  Phi : Outport
  wires:
  <DCM_b_n>/1 -> Transpose/1
  MATLAB Function1/1(Phi) -> Phi/1
  wxyz/1 -> MATLAB Function1/3(wxyz)
  axyz/1 -> MATLAB Function1/1(axyz)
  Constant/1 -> MATLAB Function1/4(dt)
  Transpose/1 -> MATLAB Function1/2(Cnb)

== system VB_RIFKF_GNSS_INS25/ER EKF/INS propogation/Init_PVQ/Horizontal_attitude ==
  note: gamma
  note: fai
  accl_mean_B_m/s_LPF : Inport  PortDimensions=3
  Magn_mean_B_guess_LPF : Inport  Port=2
  Enable : EnablePort
  Add : Sum  Inputs=+-
  Add1 : Sum
  Add2 : Sum
  Add3 : Sum
  Asin : Trigonometry  Operator=asin
  Atan2 : Trigonometry  Operator=atan2
  Data Type Conversion : DataTypeConversion  SaturateOnIntegerOverflow=off  RndMeth=Floor
  Deal with zero : Subsystem
  Degrees to Radians : simulink_extras/Transformations/Degrees to Radians
  Degrees to Radians1 : simulink_extras/Transformations/Degrees to Radians
  Demux : Demux  Outputs=3
  Divide : Product  Inputs=*/  OutDataTypeStr=single
  Gain1 : Gain  Gain=-1
  Gain2 : Gain  Gain=-1
  Hem2JPL : MATLAB Function  TreatAsAtomicUnit=on
  Hem2JPL1 : MATLAB Function  TreatAsAtomicUnit=on
  Magnetic declination : Constant  Value=param.fusion.magDeclDeg  OutDataTypeStr=single
  Magnetic declination1 : Constant  Value=param.control.MagnheadingCorrection  OutDataTypeStr=uint8
  Math Function : Math  Operator=magnitude^2  SignedPower=on
  Mux : Mux  Inputs=3
  Mux1 : Mux  Inputs=3
  Mux3 : Mux  Inputs=3
  Product : Product  Multiplication=Matrix(*)
  Quaternions to Direction Cosine Matrix : sharedtransform/Quaternions to  Direction Cosine Matrix  aMode=aMode
  Rotation Angles to Quaternions : sharedtransform/Rotation Angles to Quaternions  rotationOrder=ZYX  aMode=aMode
  Rotation Angles to Quaternions1 : sharedtransform/Rotation Angles to Quaternions  rotationOrder=ZYX  aMode=aMode
  Scope : Scope
  Scope1 : Scope
  Selector : Selector  InputPortWidth=3  IndexOptions=Index vector (dialog)  Indices=[2]  OutputSizes=1
  Selector1 : Selector  InputPortWidth=3  IndexOptions=Index vector (dialog)  Indices=[1]  OutputSizes=1
  Sqrt : Sqrt
  Sum of Elements : Sum  Inputs=+
  Switch : Switch  Threshold=0.5  SaturateOnIntegerOverflow=off  InputSameDT=off
  Terminator : Terminator
  Transpose : Math  Operator=transpose  SignedPower=on
  Trigonometric Function1 : Trigonometry  Operator=atan2
  psi_zero : Constant  Value=psi  OutDataTypeStr=single
  psi_zero1 : Constant  Value=psi0_rad  OutDataTypeStr=single
  psi_zero2 : Constant  Value=phi0_rad  OutDataTypeStr=single
  psi_zero3 : Constant  Value=gam0_rad  OutDataTypeStr=single
  quat_0 : Outport  PortDimensions=4
  wires:
  Data Type Conversion/1 -> Scope/1
  Rotation Angles to Quaternions1/1 -> Hem2JPL1/1(q)
  Switch/1 -> quat_0/1, Scope1/1
  Magnetic declination1/1 -> Switch/2, Data Type Conversion/1
  Degrees to Radians/1 -> Terminator/1
  Add1/1 -> Mux1/1
  Gain1/1 -> Mux/3, Trigonometric Function1/2
  Transpose/1 -> Product/1
  Mux3/1 -> Rotation Angles to Quaternions1/1
  Add/1 -> Mux3/1  "psi_calbymag"
  Magnetic declination/1 -> Degrees to Radians/1
  Atan2/1 -> Add/2
  Selector/1 -> Atan2/1  "magE"
  Selector1/1 -> Atan2/2  "magN"
  Product/1 -> Selector1/1, Selector/1  "magNED"
  Magn_mean_B_guess_LPF/1 -> Product/2
  Quaternions to Direction Cosine Matrix/1 -> Transpose/1
  Rotation Angles to Quaternions/1 -> Hem2JPL/1(q)  "q0_no_yaw"
  Add3/1 -> Mux3/3, Mux1/3
  Add2/1 -> Mux1/2, Mux3/2
  psi_zero/1 -> Degrees to Radians1/1
  Mux1/1 -> Rotation Angles to Quaternions/1
  Math Function/1 -> Sum of Elements/1
  Mux/1 -> Math Function/1
  Divide/1 -> Asin/1
  Sum of Elements/1 -> Sqrt/1
  Demux/3 -> Gain1/1
  Demux/2 -> Trigonometric Function1/1, Mux/1
  Demux/1 -> Mux/2, Divide/1
  Trigonometric Function1/1 -> Gain2/1
  Deal with zero/1(Out1) -> Divide/2
  Sqrt/1 -> Deal with zero/1(In1)
  accl_mean_B_m/s_LPF/1 -> Demux/1
  Hem2JPL/1(y) -> Switch/1, Quaternions to Direction Cosine Matrix/1, Switch/3
  Degrees to Radians1/1 -> Add1/2
  psi_zero1/1 -> Add1/1
  Asin/1 -> Add2/2
  psi_zero2/1 -> Add2/1
  Gain2/1 -> Add3/2
  psi_zero3/1 -> Add3/1
